simulink model "filtering"  (R2016b)
settings: Solver=VariableStepAuto  StartTime=0.0  StopTime=1093  RelTol=1e-3
libraries: simulink x3, dspfdesign x2, dsparch4 x1, simulink_extras x1, dspstat3 x1
settings Model: Creator=jadevarelle  LastModifiedBy=jadevarelle

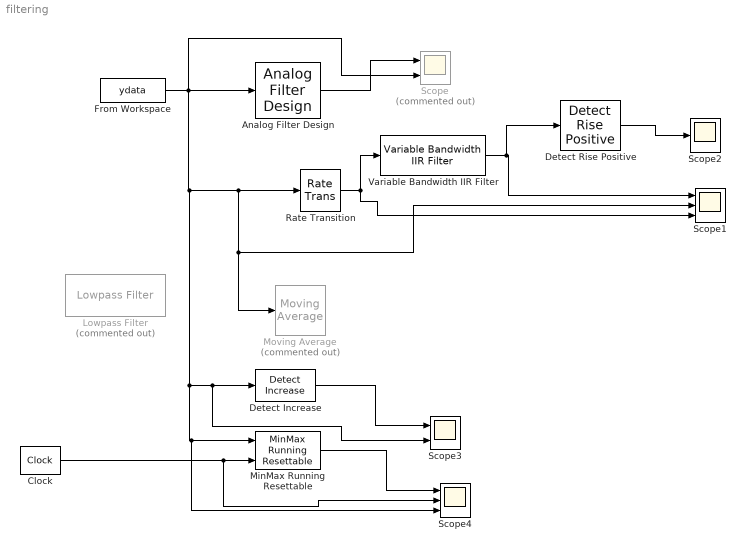
== system filtering ==
  Analog Filter Design : dsparch4/Analog Filter Design  method=Butterworth  filttype=Bandpass  N=8  Wlo=.05  Whi=2  Rp=2  Rs=40
  Clock : simulink_extras/Flip Flops/Clock  period=300
  Detect Increase : simulink/Logic and Bit Operations/Detect Increase  vinit=-.75  InputProcessing=Columns as channels (frame based)  OutDataTypeStr=boolean
  Detect Rise Positive : simulink/Logic and Bit Operations/Detect Rise Positive  vinit=-3  InputProcessing=Inherited  OutDataTypeStr=uint8
  From Workspace : FromWorkspace  VariableName=ydata  SampleTime=0
  Lowpass Filter : dspfdesign/Lowpass Filter  Commented=on  FilterType=FIR  DesignForMinimumOrder=on  FilterOrder=50  PassbandFrequency=8e3  StopbandFrequency=12e3  PassbandRipple=0.1  StopbandAttenuation=80  InheritSampleRate=off  SampleRate=44100  SimulateUsing=Interpreted execution  roundingMode=Floor  coeffsDataTypeStr=fixdt(1,16)
  MinMax Running Resettable : simulink/Math Operations/MinMax Running Resettable  Function=max  vinit=-1
  Moving Average : dspstat3/Moving Average  Commented=on  Method=Sliding window  SpecifyWindowLength=on  WindowLength=200  ForgettingFactor=0.9  SimulateUsing=Code generation
  Rate Transition : RateTransition  OutPortSampleTime=1
  Scope : Scope  Commented=on  NumInputPorts=2
  Scope1 : Scope  NumInputPorts=3
  Scope2 : Scope
  Scope3 : Scope  NumInputPorts=2
  Scope4 : Scope  NumInputPorts=3
  Variable Bandwidth IIR Filter : dspfdesign/Variable Bandwidth IIR Filter  FilterType=Lowpass  FilterOrder=8  PassbandFrequency=500  CenterFrequency=1e4  Bandwidth=2e3  PassbandRipple=.1  StopbandAttenuation=60  InheritSampleRate=off  SampleRate=44100  SimulateUsing=Code generation
  wires:
  Analog Filter Design/1 -> Scope/1
  Detect Increase/1 -> Scope3/1
  MinMax Running Resettable/1 -> Scope4/1
  Clock/1 -> Scope4/2, MinMax Running Resettable/2
  Variable Bandwidth IIR Filter/1 -> Detect Rise Positive/1, Scope1/1
  From Workspace/1 -> Scope/2, Analog Filter Design/1, Scope3/2, Detect Increase/1, Scope4/3, MinMax Running Resettable/1, Rate Transition/1, Moving Average/1, Scope1/2
  Rate Transition/1 -> Scope1/3, Variable Bandwidth IIR Filter/1
  Detect Rise Positive/1 -> Scope2/1
